simulink model "SMO_conventional"  (R2019b)
settings: Solver=VariableStepAuto  StartTime=0.0  StopTime=0.1  RelTol=1e-3
InitFcn:
  | run('MotorParamInit_1_5PMSM.m');
values from neighbouring files (symbols this model uses):
  Ibase = 2*Pbase/Vbase/3    [MotorParamInit_1_5PMSM.m]
  J = 0.01    [MotorParamInit_1_5PMSM.m]
  KpCRd = 0.104    [MotorParamInit_1_5PMSM.m]
  KpCRq = 0.104    [MotorParamInit_1_5PMSM.m]
  KpSR = 5.51    [MotorParamInit_1_5PMSM.m]
  Ld = 65.13e-3    (= 0.06513)    [MotorParamInit_1_5PMSM.m]
  LdPU = Ld/Lbase    [MotorParamInit_1_5PMSM.m]
  Lq = 120e-3    (= 0.12)    [MotorParamInit_1_5PMSM.m]
  LqPU = Lq/Lbase    [MotorParamInit_1_5PMSM.m]
  Np = 2    [MotorParamInit_1_5PMSM.m]
  PhifPU = Phif/Phibase    [MotorParamInit_1_5PMSM.m]
  Rs = 6.569    [MotorParamInit_1_5PMSM.m]
  TaoiCRd = 4e-3    (= 0.004)    [MotorParamInit_1_5PMSM.m]
  TaoiCRq = 4e-3    (= 0.004)    [MotorParamInit_1_5PMSM.m]
  TaoiSR = 80e-3    (= 0.08)    [MotorParamInit_1_5PMSM.m]
  Tctrl = 1/fctrl    (= 0.0001)    [MotorParamInit_1_5PMSM.m]
  Tembase = Pbase/Wmbase    (= 7.95774715459)    [MotorParamInit_1_5PMSM.m]
  Ts = 1e-6    (= 1e-06)    [MotorParamInit_1_5PMSM.m]
  Vbase = VN*sqrt(2)/sqrt(3)    [MotorParamInit_1_5PMSM.m]
  Wmbase = Webase/Np    (= 188.495559215)    [MotorParamInit_1_5PMSM.m]
libraries: powerlib x5, simulink x4, powerlib_extras x1
settings Model: Creator=W002220B  LastModifiedBy=W002220B

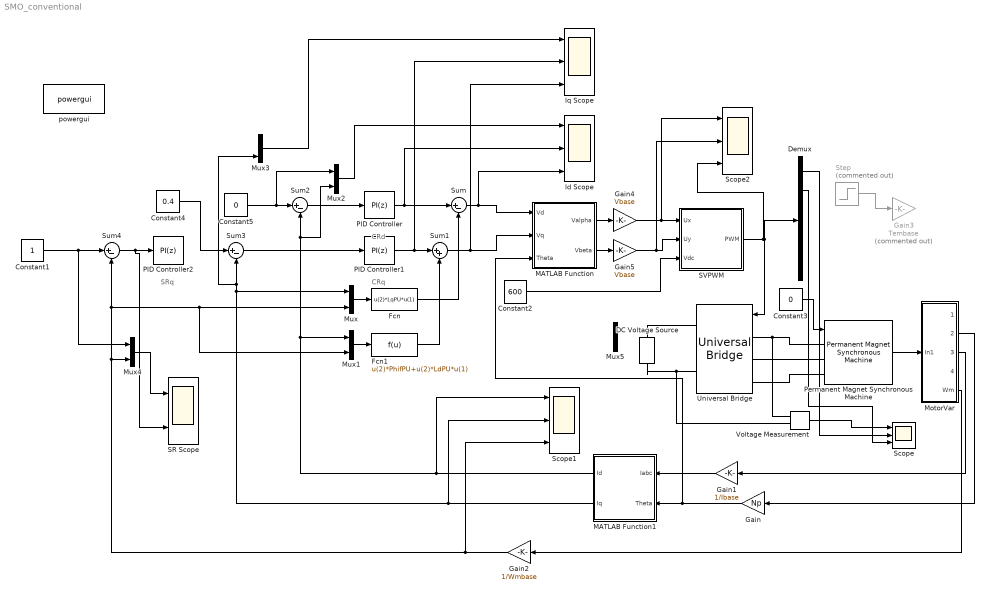
== system SMO_conventional ==
  note: CRd
  note: CRq
  note: SRq
  Constant1 : Constant
  Constant2 : Constant  Value=600
  Constant3 : Constant  Value=0
  Constant4 : Constant  Value=0.4
  Constant5 : Constant  Value=0
  DC Voltage Source : powerlib/Electrical Sources/DC Voltage Source  Amplitude=600  Measurements=None
      settings: SourceProductName=Simscape Electrical
  Demux : Demux  Outputs=6
  Fcn : Fcn  Expr=u(2)*LqPU*u(1)
  Fcn1 : Fcn  Expr=u(2)*PhifPU+u(2)*LdPU*u(1)
  Gain : Gain  Gain=Np
  Gain1 : Gain  Gain=1/Ibase
  Gain2 : Gain  Gain=1/Wmbase
  Gain3 : Gain  Commented=on  Gain=Tembase
  Gain4 : Gain  Gain=Vbase
  Gain5 : Gain  Gain=Vbase
  Id Scope : Scope  NumInputPorts=3
  Iq Scope : Scope  NumInputPorts=3
  MATLAB Function : MATLAB Function  TreatAsAtomicUnit=on
  MATLAB Function1 : MATLAB Function  TreatAsAtomicUnit=on
  MotorVar : Subsystem
  Mux{,1..5} (6 alike) : Mux  Inputs=2
  PID Controller : simulink/Continuous/PID Controller  Controller=PI  Form=Parallel  TimeDomain=Discrete-time  SampleTime=Tctrl  IntegratorMethod=Forward Euler  FilterMethod=Forward Euler  ControllerParametersSource=internal  P=KpCRd  I=KpCRd/TaoiCRd  D=0  UseFilter=on  N=100  TunerSelectOption=Transfer Function Based (PID Tuner App)  InitialConditionSource=internal  InitialConditionForIntegrator=0  InitialConditionForFilter=0  DifferentiatorICPrevScaledInput=0  ExternalReset=none  TrackingMode=off  Kt=1  LimitOutput=on  UpperSaturationLimit=0.5  LowerSaturationLimit=-0.5  LinearizeAsGain=on  AntiWindupMode=clamping  Kb=1  POutMin=[]  POutMax=[]  IOutMin=[]  IOutMax=[]  DOutMin=[]  DOutMax=[]  NOutMin=[]  NOutMax=[]  SumOutMin=[]  SumOutMax=[]  SaturationOutMin=[]  SaturationOutMax=[]  PParamMin=[]  PParamMax=[]  IParamMin=[]  IParamMax=[]  DParamMin=[]  DParamMax=[]  NParamMin=[]  NParamMax=[]  KbParamMin=[]  KbParamMax=[]  KtParamMin=[]  KtParamMax=[]  KbOutMin=[]  KbOutMax=[]  KtOutMin=[]  KtOutMax=[]  IntegratorOutMin=[]  IntegratorOutMax=[]  FilterOutMin=[]  FilterOutMax=[]  SumI1OutMin=[]  SumI1OutMax=[]  SumI2OutMin=[]  SumI2OutMax=[]  SumI3OutMin=[]  SumI3OutMax=[]  SumI4OutMin=[]  SumI4OutMax=[]  SumDOutMin=[]  SumDOutMax=[]  DifferentiatorOutMin=[]  DifferentiatorOutMax=[]  FilterDiffOutCoefMin=[]  FilterDiffOutCoefMax=[]  ReciprocalOutMin=[]  ReciprocalOutMax=[]  SumDenOutMin=[]  SumDenOutMax=[]  SumNumOutMin=[]  SumNumOutMax=[]  DivideOutMin=[]  DivideOutMax=[]  IntegratorContinuousStateAttributes=''  IntegratorStateMustResolveToSignalObject=off  IntegratorRTWStateStorageClass=Auto  FilterContinuousStateAttributes=''  FilterStateMustResolveToSignalObject=off  FilterRTWStateStorageClass=Auto  ParallelPVariant=InternalParameters  IdealPVariant=Disabled  IVariant=InternalParameters  DVariant=Disabled  IntegratorVariant=Discrete  SatVariant=Enabled  AWVariant=DiscClampingParallel  PCopyVariant=Disabled  TRVariant=Disabled  FdbkBlocksVariant=Forward  IdealPFdbkVariant=Disabled  SatFdbkVariant=Disabled  DerivativeFilterVariant=Disabled  NVariant=Disabled  NCopyVariant=Disabled_SignalSpec  FilterICVariant=Disabled  IntegratorICVariant=InternalICs  ExternalResetVariant=Disabled  TRSumVariant=Passthrough  SumFdbkVariant=Disabled  SumVariant=Sum_PI
  PID Controller1 : simulink/Continuous/PID Controller  Controller=PI  Form=Parallel  TimeDomain=Discrete-time  SampleTime=Tctrl  IntegratorMethod=Forward Euler  FilterMethod=Forward Euler  ControllerParametersSource=internal  P=KpCRq  I=KpCRq/TaoiCRq  D=0  UseFilter=on  N=100  TunerSelectOption=Transfer Function Based (PID Tuner App)  InitialConditionSource=internal  InitialConditionForIntegrator=0  InitialConditionForFilter=0  DifferentiatorICPrevScaledInput=0  ExternalReset=none  TrackingMode=off  Kt=1  LimitOutput=on  UpperSaturationLimit=0.5  LowerSaturationLimit=-0.5  LinearizeAsGain=on  AntiWindupMode=clamping  Kb=1  POutMin=[]  POutMax=[]  IOutMin=[]  IOutMax=[]  DOutMin=[]  DOutMax=[]  NOutMin=[]  NOutMax=[]  SumOutMin=[]  SumOutMax=[]  SaturationOutMin=[]  SaturationOutMax=[]  PParamMin=[]  PParamMax=[]  IParamMin=[]  IParamMax=[]  DParamMin=[]  DParamMax=[]  NParamMin=[]  NParamMax=[]  KbParamMin=[]  KbParamMax=[]  KtParamMin=[]  KtParamMax=[]  KbOutMin=[]  KbOutMax=[]  KtOutMin=[]  KtOutMax=[]  IntegratorOutMin=[]  IntegratorOutMax=[]  FilterOutMin=[]  FilterOutMax=[]  SumI1OutMin=[]  SumI1OutMax=[]  SumI2OutMin=[]  SumI2OutMax=[]  SumI3OutMin=[]  SumI3OutMax=[]  SumI4OutMin=[]  SumI4OutMax=[]  SumDOutMin=[]  SumDOutMax=[]  DifferentiatorOutMin=[]  DifferentiatorOutMax=[]  FilterDiffOutCoefMin=[]  FilterDiffOutCoefMax=[]  ReciprocalOutMin=[]  ReciprocalOutMax=[]  SumDenOutMin=[]  SumDenOutMax=[]  SumNumOutMin=[]  SumNumOutMax=[]  DivideOutMin=[]  DivideOutMax=[]  IntegratorContinuousStateAttributes=''  IntegratorStateMustResolveToSignalObject=off  IntegratorRTWStateStorageClass=Auto  FilterContinuousStateAttributes=''  FilterStateMustResolveToSignalObject=off  FilterRTWStateStorageClass=Auto  ParallelPVariant=InternalParameters  IdealPVariant=Disabled  IVariant=InternalParameters  DVariant=Disabled  IntegratorVariant=Discrete  SatVariant=Enabled  AWVariant=DiscClampingParallel  PCopyVariant=Disabled  TRVariant=Disabled  FdbkBlocksVariant=Forward  IdealPFdbkVariant=Disabled  SatFdbkVariant=Disabled  DerivativeFilterVariant=Disabled  NVariant=Disabled  NCopyVariant=Disabled_SignalSpec  FilterICVariant=Disabled  IntegratorICVariant=InternalICs  ExternalResetVariant=Disabled  TRSumVariant=Passthrough  SumFdbkVariant=Disabled  SumVariant=Sum_PI
  PID Controller2 : simulink/Continuous/PID Controller  Controller=PI  Form=Parallel  TimeDomain=Discrete-time  SampleTime=Tctrl  IntegratorMethod=Forward Euler  FilterMethod=Forward Euler  ControllerParametersSource=internal  P=KpSR  I=KpSR/TaoiSR  D=0  UseFilter=on  N=100  TunerSelectOption=Transfer Function Based (PID Tuner App)  InitialConditionSource=internal  InitialConditionForIntegrator=0  InitialConditionForFilter=0  DifferentiatorICPrevScaledInput=0  ExternalReset=none  TrackingMode=off  Kt=1  LimitOutput=on  UpperSaturationLimit=2  LowerSaturationLimit=-2  LinearizeAsGain=on  AntiWindupMode=clamping  Kb=1  POutMin=[]  POutMax=[]  IOutMin=[]  IOutMax=[]  DOutMin=[]  DOutMax=[]  NOutMin=[]  NOutMax=[]  SumOutMin=[]  SumOutMax=[]  SaturationOutMin=[]  SaturationOutMax=[]  PParamMin=[]  PParamMax=[]  IParamMin=[]  IParamMax=[]  DParamMin=[]  DParamMax=[]  NParamMin=[]  NParamMax=[]  KbParamMin=[]  KbParamMax=[]  KtParamMin=[]  KtParamMax=[]  KbOutMin=[]  KbOutMax=[]  KtOutMin=[]  KtOutMax=[]  IntegratorOutMin=[]  IntegratorOutMax=[]  FilterOutMin=[]  FilterOutMax=[]  SumI1OutMin=[]  SumI1OutMax=[]  SumI2OutMin=[]  SumI2OutMax=[]  SumI3OutMin=[]  SumI3OutMax=[]  SumI4OutMin=[]  SumI4OutMax=[]  SumDOutMin=[]  SumDOutMax=[]  DifferentiatorOutMin=[]  DifferentiatorOutMax=[]  FilterDiffOutCoefMin=[]  FilterDiffOutCoefMax=[]  ReciprocalOutMin=[]  ReciprocalOutMax=[]  SumDenOutMin=[]  SumDenOutMax=[]  SumNumOutMin=[]  SumNumOutMax=[]  DivideOutMin=[]  DivideOutMax=[]  IntegratorContinuousStateAttributes=''  IntegratorStateMustResolveToSignalObject=off  IntegratorRTWStateStorageClass=Auto  FilterContinuousStateAttributes=''  FilterStateMustResolveToSignalObject=off  FilterRTWStateStorageClass=Auto  ParallelPVariant=InternalParameters  IdealPVariant=Disabled  IVariant=InternalParameters  DVariant=Disabled  IntegratorVariant=Discrete  SatVariant=Enabled  AWVariant=DiscClampingParallel  PCopyVariant=Disabled  TRVariant=Disabled  FdbkBlocksVariant=Forward  IdealPFdbkVariant=Disabled  SatFdbkVariant=Disabled  DerivativeFilterVariant=Disabled  NVariant=Disabled  NCopyVariant=Disabled_SignalSpec  FilterICVariant=Disabled  IntegratorICVariant=InternalICs  ExternalResetVariant=Disabled  TRSumVariant=Passthrough  SumFdbkVariant=Disabled  SumVariant=Sum_PI
  Permanent Magnet Synchronous Machine : powerlib/Machines/Permanent Magnet Synchronous Machine  NbPhases=3  FluxDistribution=Sinusoidal  RotorType=Salient-pole  MechanicalLoad=Torque Tm  PresetModel=No  ShowDetailedParameters=on  MeasurementBus=off  Resistance=Rs  Inductance=8.5e-3  dqInductances=[Ld,Lq]  La=0.000395  MachineConstant=Flux linkage established by magnets (V.s)  Flux=Phif  VoltageCst=241.202  TorqueCst=1.9947  Flat=120  Mechanical=[J 0.0004924 Np 0]  PolePairs=4  InitialConditions=[0,0, 0,0]  InitialConditions5ph=[0 0 0 0 0 0]  RefAngle=Aligned with phase A axis (original Park)  IterativeDiscreteModel=Trapezoidal non iterative  TsBlock=-1  TsPowergui=0
  SR Scope : Scope  NumInputPorts=2
  SVPWM : Subsystem  mask{DT=2e-6}
      mask prompts: DT "Dead Time (s)"
  Scope : Scope  NumInputPorts=3
  Scope1 : Scope  NumInputPorts=3
  Scope2 : Scope  NumInputPorts=3
  Step : Step  Commented=on  After=0.5  SampleTime=0
  Sum{,2..4} (4 alike) : Sum  Inputs=|+-
  Sum1 : Sum  Inputs=|++
  Universal Bridge : powerlib/Power Electronics/Universal Bridge  Arms=3  SnubberResistance=1e5  SnubberCapacitance=inf  Device=MOSFET / Diodes  Ron=1e-3  Lon=0  ForwardVoltages="[  0  0  ]"  ForwardVoltage=0  GTOparameters=[ 10e-6 , 20e-6 ]  IGBTparameters=[ 1e-6 , 2e-6 ]  Measurements=None  Measurements_2=None  converterType=Rectifier
      settings: SourceProductName=Simscape Electrical
  Voltage Measurement : powerlib/Measurements/Voltage Measurement  PhasorSimulation=off  OutputType=Complex  PSBequivalent=0
      settings: SourceProductName=Simscape Electrical
  powergui : powerlib/powergui  Priority=1  SimulationMode=Discrete  SampleTime=Ts  frequency=60  Iterations=50  frequencyindice=0  Pbase=100e6  ErrMax=1e-4  UnitsV=kV  UnitsW=MW  buscounter=0  FunctionMessages=off  echomessages=off  EnableUseOfTLC=off  CurrentSourceSwitches=off  DisableSnubberDevices=off  DisableRonSwitches=off  DisableVfSwitches=off  DisplayEquations=off  AutomaticDiscreteSolvers=off  SolverType=Tustin/Backward Euler (TBE)  Interpol=off  ExternalGateDelay=off  methode=off  Ts=100  x0status=blocks  SPID=on  SwTol=0  HookPort=off  NonlinearTolerance=1e-4  nMaxIteration=100  ContinueOnMaxIteration=off  RestoreLinks=warning  ResistiveCurrentMeasurement=off  Frange=[0:2:500]  Ylog=off  Xlog=on  ShowGrid=off  save=off  variable=ZData  structure=0  ZoomFFT=off  StartTime=0.0  cycles=1  DisplayStyle=1  fundamental=60  FreqAxis=off  MaxFrequency=1000  frequencyindicesteady=1  RmsSteady=1  display=off
      settings: SourceProductName=Simscape Electrical
  wires:
  SVPWM/1(PWM) -> Universal Bridge/1, Demux/1, Scope2/3
  MATLAB Function/1(Valpha) -> Gain4/1
  Sum/1 -> Id Scope/3, MATLAB Function/1(Vd)
  Sum1/1 -> Iq Scope/3, MATLAB Function/2(Vq)
  PID Controller/1 -> Id Scope/2, Sum/1
  PID Controller1/1 -> Iq Scope/2, Sum1/1
  Sum2/1 -> PID Controller/1
  Constant5/1 -> Mux2/1, Sum2/1
  Sum3/1 -> PID Controller1/1
  Permanent Magnet Synchronous Machine/1 -> MotorVar/1(In1)
  Gain/1 -> MATLAB Function/3(Theta), MATLAB Function1/2(Theta)
  MotorVar/2(Thetam) -> Gain/1
  MATLAB Function1/1(Id) -> Scope1/1, Mux1/1, Mux2/2, Sum2/2
  MATLAB Function1/2(Iq) -> Scope1/2, Mux/1, Mux3/2, Sum3/2
  Gain1/1 -> MATLAB Function1/1(Iabc)
  MotorVar/3(Iabc) -> Gain1/1
  Constant1/1 -> Mux4/1, Sum4/1
  Sum4/1 -> SR Scope/2, PID Controller2/1
  MotorVar/5(Wm) -> Gain2/1
  Constant2/1 -> SVPWM/3(Vdc)
  Mux/1 -> Fcn/1
  Fcn/1 -> Sum/2
  Fcn1/1 -> Sum1/2
  Mux1/1 -> Fcn1/1
  MATLAB Function/2(Vbeta) -> Gain5/1
  Gain4/1 -> Scope2/1, SVPWM/1(Ux)
  Gain5/1 -> Scope2/2, SVPWM/2(Uy)
  Mux2/1 -> Id Scope/1
  Mux3/1 -> Iq Scope/1
  Mux4/1 -> SR Scope/1
  Gain2/1 -> Scope1/3, Mux4/2, Mux/2, Mux1/2, Sum4/2
  Step/1 -> Gain3/1
  Constant3/1 -> Permanent Magnet Synchronous Machine/1
  Voltage Measurement/1 -> Scope/1
  Demux/1 -> Scope/2
  Demux/2 -> Scope/3
  Constant4/1 -> Sum3/1
  connections:
  Permanent Magnet Synchronous Machine/LConn2 -- Universal Bridge/LConn2
  Permanent Magnet Synchronous Machine/LConn3 -- Universal Bridge/LConn3
  Permanent Magnet Synchronous Machine/LConn1 -- Voltage Measurement/LConn1 -- Universal Bridge/LConn1
  DC Voltage Source/LConn1 -- Voltage Measurement/LConn2 -- Universal Bridge/RConn2
  DC Voltage Source/RConn1 -- Universal Bridge/RConn1

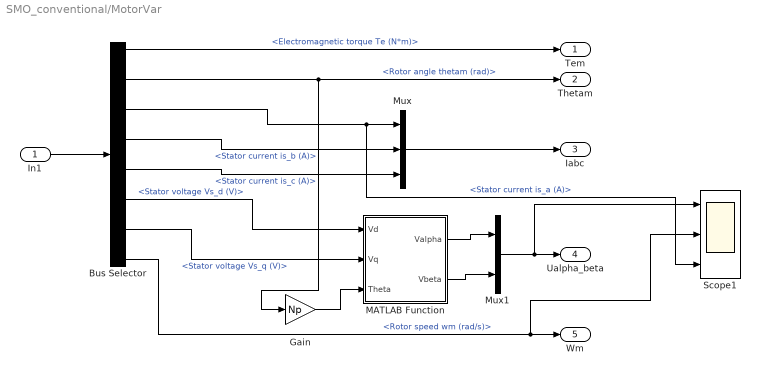
== system SMO_conventional/MotorVar ==
  In1 : Inport
  Bus Selector : BusSelector  OutputSignals=Electromagnetic torque Te (N*m),Rotor angle thetam (rad),Stator current is_a (A),Stator current is_b (A),Stator current is_c (A),Stator voltage Vs_d (V),Stator voltage Vs_q (V),Rotor speed wm (rad/s)
  Gain : Gain  Gain=Np
  MATLAB Function : MATLAB Function  TreatAsAtomicUnit=on
  Mux : Mux  Inputs=3
  Mux1 : Mux  Inputs=2
  Scope1 : Scope  NumInputPorts=3
  Tem : Outport
  Thetam : Outport  Port=2
  Iabc : Outport  Port=3
  Ualpha_beta : Outport  Port=4
  Wm : Outport  Port=5
  wires:
  In1/1 -> Bus Selector/1
  Bus Selector/1 -> Tem/1  "<Electromagnetic torque Te (N*m)>"
  Bus Selector/2 -> Gain/1, Thetam/1  "<Rotor angle thetam (rad)>"
  Bus Selector/3 -> Scope1/3, Mux/1  "<Stator current is_a (A)>"
  Mux/1 -> Iabc/1
  Bus Selector/6 -> MATLAB Function/1(Vd)  "<Stator voltage Vs_d (V)>"
  Bus Selector/7 -> MATLAB Function/2(Vq)  "<Stator voltage Vs_q (V)>"
  Gain/1 -> MATLAB Function/3(Theta)
  MATLAB Function/1(Valpha) -> Mux1/1
  MATLAB Function/2(Vbeta) -> Mux1/2
  Mux1/1 -> Scope1/1, Ualpha_beta/1
  Bus Selector/8 -> Scope1/2, Wm/1  "<Rotor speed wm (rad/s)>"
  Bus Selector/4 -> Mux/2  "<Stator current is_b (A)>"
  Bus Selector/5 -> Mux/3  "<Stator current is_c (A)>"

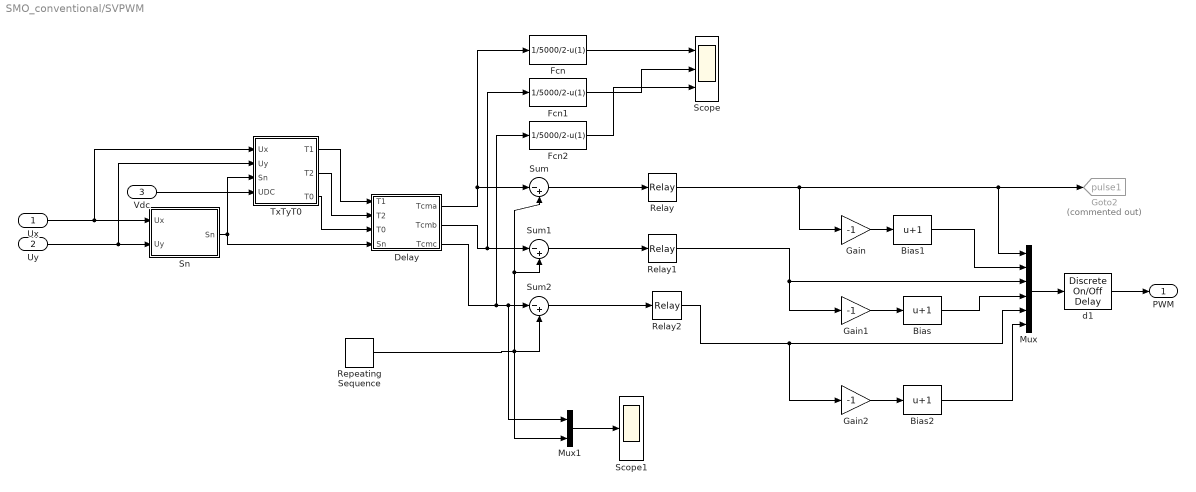
== system SMO_conventional/SVPWM ==
  Ux : Inport
  Uy : Inport  Port=2
  Vdc : Inport  Port=3
  Bias : Bias  Bias=1
  Bias1 : Bias  Bias=1
  Bias2 : Bias  Bias=1
  Delay : MATLAB Function  TreatAsAtomicUnit=on
  Fcn : Fcn  Expr=1/5000/2-u(1)
  Fcn1 : Fcn  Expr=1/5000/2-u(1)
  Fcn2 : Fcn  Expr=1/5000/2-u(1)
  Gain : Gain  Gain=-1
  Gain1 : Gain  Gain=-1
  Gain2 : Gain  Gain=-1
  Goto2 : Goto  Commented=on  GotoTag=pulse1  TagVisibility=global
  Mux : Mux  Inputs=6
  Mux1 : Mux  Inputs=2
  Relay : Relay  OnSwitchValue=0  OffSwitchValue=0
  Relay1 : Relay  OnSwitchValue=0  OffSwitchValue=0
  Relay2 : Relay  OnSwitchValue=0  OffSwitchValue=0
  Repeating Sequence : simulink/Sources/Repeating Sequence  rep_seq_t=[0 1/5000/2 1/5000]  rep_seq_y=[0 1/5000/2 0]
  Scope : Scope  NumInputPorts=3
  Scope1 : Scope
  Sn : MATLAB Function  TreatAsAtomicUnit=on
  Sum : Sum  Inputs=|-+
  Sum1 : Sum  Inputs=|-+
  Sum2 : Sum  Inputs=|-+
  TxTyT0 : MATLAB Function  TreatAsAtomicUnit=on
  d1 : powerlib_extras/Discrete  Control Blocks/Discrete On//Off Delay  type_delay=On delay  delay=DT  ic=0  Ts=Ts
      settings: SourceProductName=Simscape Electrical  SourceProductBaseCode=PS
  PWM : Outport
  wires:
  Delay/1(Tcma) -> Fcn/1, Sum/1
  Delay/2(Tcmb) -> Fcn1/1, Sum1/1
  Delay/3(Tcmc) -> Fcn2/1, Mux1/1, Sum2/1
  Repeating Sequence/1 -> Mux1/2, Sum2/2, Sum/2, Sum1/2
  Sum/1 -> Relay/1
  Sum2/1 -> Relay2/1
  Sum1/1 -> Relay1/1
  Relay1/1 -> Gain1/1, Mux/3
  Relay2/1 -> Gain2/1, Mux/5
  Sn/1(Sn) -> TxTyT0/3(Sn), Delay/4(Sn)
  TxTyT0/1(T1) -> Delay/1(T1)
  TxTyT0/2(T2) -> Delay/2(T2)
  TxTyT0/3(T0) -> Delay/3(T0)
  Gain1/1 -> Bias/1
  Gain/1 -> Bias1/1
  Gain2/1 -> Bias2/1
  Relay/1 -> Gain/1, Mux/1, Goto2/1
  Ux/1 -> Sn/1(Ux), TxTyT0/1(Ux)
  Uy/1 -> Sn/2(Uy), TxTyT0/2(Uy)
  Vdc/1 -> TxTyT0/4(UDC)
  Bias1/1 -> Mux/2
  Bias/1 -> Mux/4
  Bias2/1 -> Mux/6
  d1/1 -> PWM/1
  Mux/1 -> d1/1
  Fcn/1 -> Scope/1
  Fcn1/1 -> Scope/2
  Fcn2/1 -> Scope/3
  Mux1/1 -> Scope1/1

== matlab function SMO_conventional/SVPWM/Sn ==
  data: Sn output; Ux input; Uy input
function Sn = S(Ux,Uy)
theta=atan2(Uy,Ux)*180/pi;
if theta>=0&&theta<60
    Sn=1;
elseif theta>=60&&theta<120
    Sn=2;
elseif theta>=120&&theta<180
    Sn=3;
elseif theta>=-180&&theta<-120
    Sn=4;
elseif theta>=-120&&theta<-60
    Sn=5;
else Sn=6;
end

== matlab function SMO_conventional/MATLAB Function ==
  data: Valpha output; Vd input; Vbeta output; Vq input; Theta input
function [Valpha, Vbeta] = fcn(Vd, Vq, Theta)
%#codegen

Valpha = Vd*cos(Theta) - Vq*sin(Theta);
Vbeta  = Vd*sin(Theta) + Vq*cos(Theta);

== matlab function SMO_conventional/SVPWM/TxTyT0 ==
  data: Ux input; Uy input; Sn input; T1 output; T2 output; T0 output; UDC input
function [T1,T2,T0]=T(Ux,Uy,Sn,UDC)
Ts=1/5000;
Udc=UDC;

X=sqrt(3)*Ts/Udc*Uy;
Y=sqrt(3)*Ts/2/Udc*(sqrt(3)*Ux+Uy);
Z=sqrt(3)*Ts/2/Udc*(-sqrt(3)*Ux+Uy);

if Sn==1
    T1=-Z;T2=X;
elseif Sn==2;
    T1=Z;T2=Y;
elseif Sn==3;
    T1=X;T2=-Y;
elseif Sn==4;
    T1=-X;T2=Z;
elseif Sn==5;
    T1=-Y;T2=-Z;
else T1=Y;T2=-X;
end
    
if T1+T2>Ts
    a=T1;b=T2;
    T1=a*Ts/(a+b);
    T2=b*Ts/(a+b);
end

T0=Ts-T1-T2;

== matlab function SMO_conventional/SVPWM/Delay ==
  data: T1 input; T2 input; T0 input; Tcma output; Tcmb output; Tcmc output; Sn input
function [Tcma,Tcmb,Tcmc]=D(T1,T2,T0,Sn)
T=1/5000;
ton1=0.25*T0;
ton2=ton1+T1/2;
ton3=ton2+T2/2;
if Sn==1
    Tcma=ton1;Tcmb=ton2;Tcmc=ton3;
elseif Sn==2;
    Tcma=ton2;Tcmb=ton1;Tcmc=ton3;
elseif Sn==3;
    Tcma=ton3;Tcmb=ton1;Tcmc=ton2;
elseif Sn==4;
    Tcma=ton3;Tcmb=ton2;Tcmc=ton1;
elseif Sn==5;
    Tcma=ton2;Tcmb=ton3;Tcmc=ton1;
else Tcma=ton1;Tcmb=ton3;Tcmc=ton2;
end

== matlab function SMO_conventional/MotorVar/MATLAB Function ==
  data: Valpha output; Vd input; Vbeta output; Vq input; Theta input
function [Valpha, Vbeta] = fcn(Vd, Vq, Theta)
%#codegen

Valpha = Vd*cos(Theta) - Vq*sin(Theta);
Vbeta  = Vd*sin(Theta) + Vq*cos(Theta);

== matlab function SMO_conventional/MATLAB Function1 ==
  data: Id output; Iabc input; Iq output; Theta input
function [Id, Iq] = fcn(Iabc,Theta)
%#codegen

Id =  Iabc(1)*cos(Theta) + Iabc(2)*cos(Theta-2*pi/3) + Iabc(3)*cos(Theta+2*pi/3);
Iq  = -Iabc(1)*sin(Theta) - Iabc(2)*sin(Theta-2*pi/3) - Iabc(3)*sin(Theta+2*pi/3);
Id = Id*2/3;
Iq = Iq*2/3;
